simulink model "capitol4pb4"  (R2013a)
settings: Solver=ode45  StartTime=0.0  StopTime=43800  RelTol=1e-3
undefined symbols (not defined in the file): des, gcbh
settings Model: Creator=user  LastModifiedBy=user

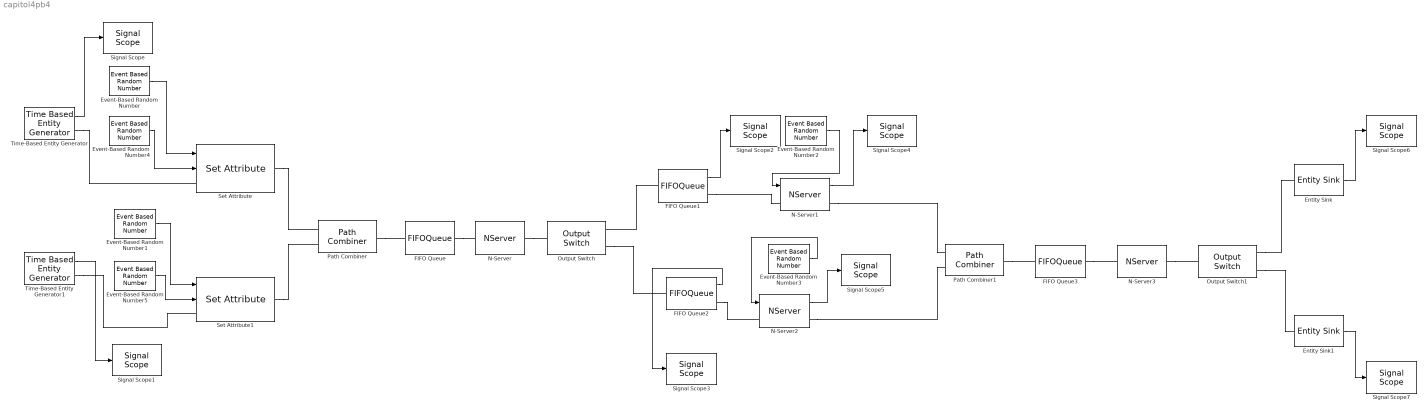
== system capitol4pb4 ==
  Entity Sink : EntitySink  StatNumberArrived=on
  Entity Sink1 : EntitySink  StatNumberArrived=on
  Event-Based Random Number : EventBasedRandomNumber  Distribution=Uniform  minUnif=13  maxUnif=27  Seed=3242344
  Event-Based Random Number1 : EventBasedRandomNumber  Distribution=Uniform  minUnif=33  maxUnif=57  Seed=52487
  Event-Based Random Number2 : EventBasedRandomNumber  Distribution=Uniform  minUnif=600  maxUnif=840
  Event-Based Random Number3 : EventBasedRandomNumber  Distribution=Uniform  minUnif=960  maxUnif=1440
  Event-Based Random Number4 : EventBasedRandomNumber  Distribution=Uniform  minUnif=20  maxUnif=30
  Event-Based Random Number5 : EventBasedRandomNumber  Distribution=Uniform  minUnif=25  maxUnif=35
  FIFO Queue : FIFOQueue
  FIFO Queue1 : FIFOQueue  StatNumberDeparted=on
  FIFO Queue2 : FIFOQueue  StatNumberDeparted=on
  FIFO Queue3 : FIFOQueue
  N-Server : NServer  NumberOfServers=2  ServiceTimeFrom=Attribute  AttributeName=Intrare
  N-Server1 : NServer  NumberOfServers=6  ServiceTimeFrom=Signal port t  StatNumberDeparted=on
  N-Server2 : NServer  NumberOfServers=3  ServiceTimeFrom=Signal port t  StatNumberDeparted=on
  N-Server3 : NServer  NumberOfServers=2  ServiceTimeFrom=Attribute  AttributeName=Iesire
  Output Switch : OutputSwitch  NumberOutputPorts=2  SwitchingCriterion=From attribute  AttributeName=Nava
  Output Switch1 : OutputSwitch  NumberOutputPorts=2  SwitchingCriterion=From attribute  AttributeName=Nava
  Path Combiner : PathCombiner  NumberInputPorts=2
  Path Combiner1 : PathCombiner  NumberInputPorts=2
  Set Attribute : SetAttribute  AttributeName=Nava|Intrare|Iesire  AttributeFrom=Dialog|Signal port|Signal port  AttributeValue=1|1|1  AttributeTreatAsVector=1|1|1  EvaluatedAttributeValue={ 1;[];[]}
      settings: InputPortMap=u1,u2
  Set Attribute1 : SetAttribute  AttributeName=Nava|Intrare|Iesire  AttributeFrom=Dialog|Signal port|Signal port  AttributeValue=2|1|1  AttributeTreatAsVector=1|1|1  EvaluatedAttributeValue={ 2;[];[]}
      settings: InputPortMap=u1,u2
  Signal Scope{,1..5} (6 alike) : SignalScope  LoadFcn=des.scope.CallbackSupport('seLoadFcn',gcbh)  StartFcn=des.scope.CallbackSupport('seStartFcn',gcbh)  StopFcn=des.scope.CallbackSupport('seStopFcn',gcbh)
      settings: CopyFcn=des.scope.CallbackSupport('seCopyFcn',gcbh)  DeleteFcn=des.scope.CallbackSupport('seDeleteFcn',gcbh)  PreSaveFcn=des.scope.CallbackSupport('sePreSaveFcn',gcbh)  NameChangeFcn=des.scope.CallbackSupport('seNameChangeFcn',gcbh)  OpenFcn=des.scope.CallbackSupport('seOpenFcn',gcbh)
  Signal Scope6 : SignalScope  LoadFcn=des.scope.CallbackSupport('seLoadFcn',gcbh)  StartFcn=des.scope.CallbackSupport('seStartFcn',gcbh)  StopFcn=des.scope.CallbackSupport('seStopFcn',gcbh)  XMin=-431.153574206018  XMax=43546.5109948078
      settings: CopyFcn=des.scope.CallbackSupport('seCopyFcn',gcbh)  DeleteFcn=des.scope.CallbackSupport('seDeleteFcn',gcbh)  PreSaveFcn=des.scope.CallbackSupport('sePreSaveFcn',gcbh)  NameChangeFcn=des.scope.CallbackSupport('seNameChangeFcn',gcbh)  OpenFcn=des.scope.CallbackSupport('seOpenFcn',gcbh)  YMin=-3.75  YMax=378.75
  Signal Scope7 : SignalScope  LoadFcn=des.scope.CallbackSupport('seLoadFcn',gcbh)  StartFcn=des.scope.CallbackSupport('seStartFcn',gcbh)  StopFcn=des.scope.CallbackSupport('seStopFcn',gcbh)  XMax=81920
      settings: CopyFcn=des.scope.CallbackSupport('seCopyFcn',gcbh)  DeleteFcn=des.scope.CallbackSupport('seDeleteFcn',gcbh)  PreSaveFcn=des.scope.CallbackSupport('sePreSaveFcn',gcbh)  NameChangeFcn=des.scope.CallbackSupport('seNameChangeFcn',gcbh)  OpenFcn=des.scope.CallbackSupport('seOpenFcn',gcbh)  YMax=320
  Time-Based Entity Generator : TimeBasedEntityGenerator  Distribution=Uniform  Period=0.5  InitialSeed=23423  Minimum=100  Maximum=130  StatNumberDeparted=on
  Time-Based Entity Generator1 : TimeBasedEntityGenerator  Distribution=Uniform  InitialSeed=2355346  Minimum=193  Maximum=207  StatNumberDeparted=on
  wires:
  Time-Based Entity Generator/1 -> Signal Scope/1
  Event-Based Random Number/1 -> Set Attribute/1
  Time-Based Entity Generator1/1 -> Signal Scope1/1
  Event-Based Random Number1/1 -> Set Attribute1/1
  FIFO Queue1/1 -> Signal Scope2/1
  FIFO Queue2/1 -> Signal Scope3/1
  Event-Based Random Number2/1 -> N-Server1/1
  Event-Based Random Number3/1 -> N-Server2/1
  N-Server1/1 -> Signal Scope4/1
  N-Server2/1 -> Signal Scope5/1
  Entity Sink/1 -> Signal Scope6/1
  Entity Sink1/1 -> Signal Scope7/1
  Event-Based Random Number4/1 -> Set Attribute/2
  Event-Based Random Number5/1 -> Set Attribute1/2
  connections:
  Time-Based Entity Generator/RConn1 -- Set Attribute/LConn1
  Set Attribute/RConn1 -- Path Combiner/LConn1
  Set Attribute1/RConn1 -- Path Combiner/LConn2
  Path Combiner/RConn1 -- FIFO Queue/LConn1
  FIFO Queue/RConn1 -- N-Server/LConn1
  N-Server/RConn1 -- Output Switch/LConn1
  FIFO Queue1/LConn1 -- Output Switch/RConn1
  Output Switch/RConn2 -- FIFO Queue2/LConn1
  FIFO Queue1/RConn1 -- N-Server1/LConn1
  FIFO Queue2/RConn1 -- N-Server2/LConn1
  N-Server1/RConn1 -- Path Combiner1/LConn1
  N-Server2/RConn1 -- Path Combiner1/LConn2
  Path Combiner1/RConn1 -- FIFO Queue3/LConn1
  FIFO Queue3/RConn1 -- N-Server3/LConn1
  N-Server3/RConn1 -- Output Switch1/LConn1
  Output Switch1/RConn1 -- Entity Sink/LConn1
  Output Switch1/RConn2 -- Entity Sink1/LConn1
  Time-Based Entity Generator1/RConn1 -- Set Attribute1/LConn1
